simulink model "sampleModel1955_4_sub"  (R2023a)
settings: Solver=VariableStepAuto  StartTime=0.0  StopTime=10.0  RelTol=1e-3
libraries: simulink x6, hdlsllib x4
settings Model: Creator=user1  LastModifiedBy=user1
settings OptimizationCC: BlockReduction=off  ConditionallyExecuteInputs=off

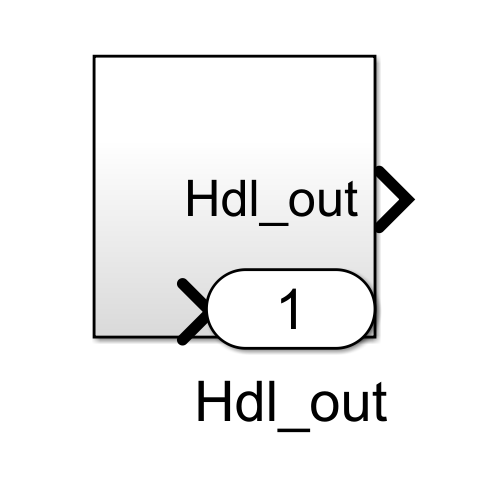
[thumbnail: Simulink's stored preview of the top-level diagram]
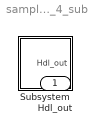
== system sampleModel1955_4_sub ==
  Subsystem : Subsystem
  Hdl_out : Outport  OutDataTypeStr=uint8

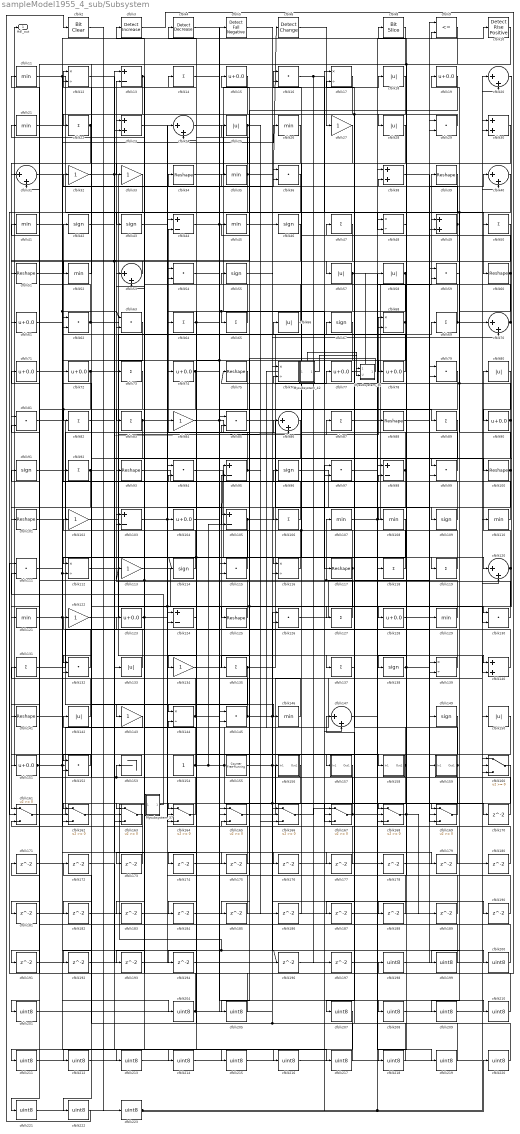
== system sampleModel1955_4_sub/Subsystem ==
  Mysubsystem_30 : Subsystem  TreatAsAtomicUnit=on  RTWFcnName=Mysubsystem_30
      settings: RTWFcnNameOpts=User specified  RTWFileNameOpts=Use function name
  Mysubsystem_37 : Subsystem  TreatAsAtomicUnit=on  RTWFcnName=Mysubsystem_37
      settings: RTWFcnNameOpts=User specified  RTWFileNameOpts=Use function name
  Mysubsystem_42 : Subsystem  TreatAsAtomicUnit=on  RTWFcnName=Mysubsystem_42
      settings: RTWFcnNameOpts=User specified  RTWFileNameOpts=Use function name
  cfblk10 : hdlsllib/Logic and Bit Operations/Detect Rise Positive  vinit=0  OutDataTypeStr=uint8
  cfblk{34,39,51,60,75,88,93,100..101,117,125,141} (12 alike) : Reshape
  cfblk{27,32..33,84,102,113,122,134,143} (9 alike) : Gain  OutDataTypeStr=uint8
  cfblk{13,44,95,98,103,105,124} (7 alike) : Sum  Inputs=+-  OutDataTypeStr=uint8
  cfblk{15,19,61,71..72,74,77..78,90,104,123,128,151} (13 alike) : Bias  Bias=0.0  SaturateOnIntegerOverflow=off
  cfblk{14,22,47,50,64..65,69,73,82..83,87,89,92,106,118..119,127,131,135,137} (20 alike) : Sum  Inputs=+  OutDataTypeStr=uint8
  cfblk{11,21,26,35,41,45,52,107..108,110,121,129,146} (13 alike) : MinMax  OutDataTypeStr=uint8
  cfblk{42..43,46,55,67,91,96,109,114,138,149} (11 alike) : Signum
  cfblk{16,29,36,54,59,62..63,79,81,85,94,97,99,111,115,126,130,132,145,152} (20 alike) : DotProduct  OutDataTypeStr=uint8
  cfblk{12,17,48,68,76,112,116,139,144} (9 alike) : Product  Inputs=*/  OutDataTypeStr=uint8  RndMeth=Zero  SaturateOnIntegerOverflow=on
  cfblk{20,24,31,40,53,70,86,120,147} (9 alike) : Sum  Inputs=|++  OutDataTypeStr=uint8
  cfblk{18,25,28,57..58,66,80,133,142,150} (10 alike) : Abs  OutDataTypeStr=uint8  SaturateOnIntegerOverflow=off
  cfblk{23,30,38,49,140} (5 alike) : Sum  OutDataTypeStr=uint8
  cfblk153 : Terminator
  cfblk154 : Constant  OutDataTypeStr=uint8  SampleTime=-1
  cfblk155 : hdlsllib/Sources/Counter Free-Running  NumBits=16  tsamp=-1
  cfblk156 : Subsystem
      settings: LibrarySourceBlock=|
      | hdlsllib/Ports &
      | Subsystems/Subsystem
  cfblk157 : Subsystem
      settings: LibrarySourceBlock=|
      | hdlsllib/Ports &
      | Subsystems/Subsystem
  cfblk158 : Subsystem
      settings: LibrarySourceBlock=|
      | hdlsllib/Ports &
      | Subsystems/Subsystem
  cfblk159 : Subsystem
      settings: LibrarySourceBlock=|
      | hdlsllib/Ports &
      | Subsystems/Subsystem
  cfblk{160..169} (10 alike) : Switch  OutDataTypeStr=uint8  SaturateOnIntegerOverflow=off  InputSameDT=off
  cfblk{170..194,196..197} (27 alike) : Delay  SampleTime=1
  cfblk{198..201,204..205,207..223} (23 alike) : DataTypeConversion  OutDataTypeStr=uint8  SaturateOnIntegerOverflow=off  RndMeth=Floor
  cfblk2 : simulink/Logic and Bit Operations/Bit Clear  iBit=0
      settings: LibrarySourceBlock=|
      | hdlsllib/Logic and Bit
      | Operations/Bit Clear
  cfblk3 : simulink/Logic and Bit Operations/Detect Increase  vinit=0.0  OutDataTypeStr=uint8
      settings: LibrarySourceBlock=|
      | hdlsllib/Logic and Bit
      | Operations/Detect
      | Increase
  cfblk4 : simulink/Logic and Bit Operations/Detect Decrease  vinit=0.0  OutDataTypeStr=uint8
      settings: LibrarySourceBlock=|
      | hdlsllib/Logic and Bit
      | Operations/Detect
      | Decrease
  cfblk5 : hdlsllib/Logic and Bit Operations/Detect Fall Negative  vinit=0  OutDataTypeStr=uint8
  cfblk6 : simulink/Logic and Bit Operations/Detect Change  vinit=0  OutDataTypeStr=uint8
      settings: LibrarySourceBlock=|
      | hdlsllib/Logic and Bit
      | Operations/Detect
      | Change
  cfblk8 : hdlsllib/Logic and Bit Operations/Bit Slice  lidx=7  ridx=0
  cfblk9 : RelationalOperator  Operator=<=  OutDataTypeStr=boolean  InputSameDT=off
  Hdl_out : Outport  OutDataTypeStr=uint8
  wires:
  cfblk81/1 -> cfblk143/1
  cfblk29/1 -> cfblk28/1
  cfblk77/1 -> cfblk58/1
  cfblk144/1 -> cfblk179/1, cfblk102/1
  cfblk135/1 -> cfblk162/1, cfblk77/1
  cfblk92/1 -> cfblk191/1, cfblk100/1
  cfblk143/1 -> cfblk142/1
  cfblk19/1 -> cfblk161/1
  cfblk105/1 -> cfblk69/1, cfblk184/1, cfblk114/1
  cfblk83/1 -> cfblk192/1, cfblk67/1
  cfblk20/1 -> cfblk99/1
  cfblk95/1 -> cfblk186/1, cfblk44/2
  cfblk26/1 -> cfblk81/1
  cfblk164/1 -> cfblk122/1
  cfblk127/1 -> cfblk34/1, cfblk107/1
  cfblk32/1 -> cfblk86/2, cfblk137/1
  cfblk107/1 -> cfblk9/2, cfblk39/1
  cfblk6/1 -> cfblk27/1
  cfblk122/1 -> cfblk66/1
  cfblk106/1 -> cfblk42/1
  cfblk27/1 -> cfblk106/1
  cfblk48/1 -> cfblk138/1
  cfblk130/1 -> cfblk13/2
  cfblk169/1 -> cfblk91/1
  cfblk57/1 -> cfblk169/2, cfblk164/2, cfblk65/1
  cfblk96/1 -> cfblk139/2
  cfblk34/1 -> cfblk18/1
  cfblk73/1 -> cfblk101/1, cfblk82/1
  cfblk44/1 -> cfblk140/1, cfblk76/1
  cfblk28/1 -> cfblk33/1
  cfblk9/1 -> cfblk218/1, cfblk212/1
  cfblk161/1 -> cfblk118/1
  cfblk116/1 -> cfblk72/1
  cfblk112/1 -> cfblk87/1
  cfblk45/1 -> cfblk46/1
  cfblk162/1 -> cfblk73/1
  cfblk113/1 -> cfblk128/1
  cfblk94/1 -> cfblk120/1
  cfblk43/1 -> cfblk124/1
  cfblk101/1 -> cfblk17/1
  cfblk147/1 -> cfblk219/1
  cfblk25/1 -> cfblk166/3, cfblk61/1
  cfblk151/1 -> Hdl_out/1, cfblk36/2, cfblk133/1
  cfblk90/1 -> cfblk199/1, cfblk49/1, cfblk75/1
  cfblk10/1 -> cfblk52/1
  cfblk24/1 -> cfblk117/1
  cfblk35/1 -> cfblk221/1, cfblk12/2, cfblk6/1
  cfblk74/1 -> cfblk201/1, cfblk157/1(In1)
  cfblk49/1 -> cfblk12/1, cfblk108/1
  cfblk118/1 -> cfblk76/2, cfblk95/1
  cfblk168/1 -> cfblk189/1, cfblk188/1
  cfblk2/1 -> cfblk223/1
  cfblk120/1 -> cfblk164/3, cfblk80/1
  cfblk137/1 -> cfblk17/2
  cfblk11/1 -> cfblk216/1, cfblk60/1
  cfblk36/1 -> cfblk163/1
  cfblk140/1 -> cfblk14/1
  cfblk89/1 -> cfblk116/1
  cfblk78/1 -> cfblk15/1
  cfblk121/1 -> cfblk35/1, cfblk196/1, Mysubsystem_37/1(In1)
  cfblk91/1 -> cfblk74/1
  cfblk134/1 -> cfblk95/2
  cfblk129/1 -> cfblk47/1
  cfblk123/1 -> cfblk127/1, cfblk23/1
  cfblk50/1 -> cfblk57/1
  cfblk117/1 -> cfblk53/1, cfblk132/1, cfblk135/1
  cfblk84/1 -> cfblk177/1, cfblk86/1
  cfblk110/1 -> cfblk54/1
  cfblk23/1 -> cfblk105/1
  cfblk39/1 -> cfblk161/2
  cfblk18/1 -> cfblk187/1, cfblk132/2
  cfblk62/1 -> cfblk31/2, cfblk85/1
  cfblk146/1 -> cfblk53/2
  cfblk40/1 -> cfblk49/2, cfblk169/1
  cfblk17/1 -> cfblk22/1
  cfblk159/1(Out1) -> cfblk168/2, cfblk93/1
  cfblk22/1 -> cfblk182/1, cfblk181/1
  cfblk154/1 -> cfblk113/1, cfblk103/1, cfblk105/2, cfblk169/3, Mysubsystem_42/1(In1)
  cfblk38/1 -> cfblk159/1(In1)
  cfblk52/1 -> cfblk32/1
  cfblk87/1 -> cfblk29/1
  cfblk128/1 -> cfblk149/1
  cfblk93/1 -> cfblk98/2
  cfblk155/1 -> cfblk167/3, cfblk168/1
  cfblk138/1 -> cfblk170/1, cfblk38/2
  cfblk99/1 -> cfblk68/1
  cfblk55/1 -> cfblk70/2
  cfblk47/1 -> cfblk163/2, cfblk121/1
  cfblk59/1 -> cfblk109/1
  cfblk145/1 -> cfblk123/1, cfblk79/2, cfblk190/1, cfblk168/3
  cfblk53/1 -> cfblk51/1
  cfblk131/1 -> cfblk29/2
  cfblk46/1 -> cfblk145/2
  cfblk156/1(Out1) -> cfblk165/2
  cfblk58/1 -> cfblk194/1, cfblk78/1
  cfblk69/1 -> cfblk40/2, cfblk8/1
  cfblk165/1 -> cfblk20/1
  cfblk163/1 -> cfblk161/3
  cfblk100/1 -> cfblk19/1, cfblk152/1
  cfblk115/1 -> cfblk24/2
  cfblk158/1(Out1) -> cfblk162/2, cfblk64/1
  cfblk64/1 -> cfblk140/2, cfblk4/1
  cfblk51/1 -> cfblk152/2
  cfblk65/1 -> cfblk55/1
  cfblk139/1 -> cfblk45/1
  cfblk60/1 -> cfblk209/1, cfblk36/1
  cfblk68/1 -> cfblk134/1, cfblk16/1
  cfblk102/1 -> cfblk124/2
  cfblk167/1 -> cfblk59/2, cfblk92/1, cfblk153/1
  cfblk72/1 -> cfblk119/1, cfblk141/1
  cfblk141/1 -> cfblk94/2
  cfblk132/1 -> cfblk11/1
  cfblk125/1 -> cfblk41/1
  cfblk13/1 -> cfblk23/2, cfblk83/1
  cfblk33/1 -> cfblk43/1
  cfblk14/1 -> cfblk89/1
  cfblk111/1 -> cfblk204/1
  cfblk108/1 -> cfblk112/1
  cfblk66/1 -> cfblk21/1
  cfblk42/1 -> cfblk50/1
  cfblk71/1 -> cfblk10/1
  cfblk82/1 -> cfblk144/1
  cfblk85/1 -> cfblk129/1
  cfblk133/1 -> cfblk81/2
  cfblk109/1 -> cfblk96/1
  cfblk79/1 -> cfblk125/1
  cfblk41/1 -> cfblk116/2
  cfblk70/1 -> cfblk130/1, cfblk25/1
  cfblk88/1 -> cfblk40/1
  cfblk80/1 -> cfblk90/1
  cfblk8/1 -> cfblk31/1
  cfblk103/1 -> cfblk104/1, cfblk130/2, cfblk146/1
  cfblk104/1 -> cfblk88/1
  cfblk152/1 -> cfblk151/1
  cfblk119/1 -> cfblk84/1
  cfblk54/1 -> cfblk126/2
  cfblk61/1 -> cfblk26/1
  cfblk16/1 -> cfblk197/1, cfblk48/2
  cfblk166/1 -> cfblk167/1
  cfblk31/1 -> cfblk158/1(In1), cfblk63/1
  cfblk67/1 -> cfblk115/2, cfblk164/1
  cfblk126/1 -> cfblk9/1
  cfblk114/1 -> cfblk63/2
  cfblk142/1 -> cfblk131/1
  cfblk63/1 -> cfblk162/3, cfblk112/2
  cfblk98/1 -> cfblk163/3, cfblk62/2
  cfblk170/1 -> cfblk48/1
  cfblk75/1 -> cfblk173/1
  cfblk173/1 -> cfblk62/1
  cfblk150/1 -> cfblk174/1
  cfblk174/1 -> cfblk167/2
  cfblk12/1 -> cfblk175/1
  cfblk175/1 -> cfblk94/1
  cfblk21/1 -> cfblk176/1
  cfblk176/1 -> cfblk120/2
  cfblk177/1 -> cfblk165/1
  cfblk178/1 -> cfblk79/1
  cfblk179/1 -> cfblk139/1
  cfblk180/1 -> cfblk165/3
  cfblk181/1 -> cfblk59/1
  cfblk182/1 -> cfblk166/2
  cfblk157/1(Out1) -> cfblk183/1
  cfblk183/1 -> cfblk98/1
  cfblk184/1 -> cfblk166/1
  cfblk185/1 -> cfblk44/1
  cfblk186/1 -> cfblk16/2
  cfblk187/1 -> cfblk38/1
  cfblk188/1 -> cfblk145/1
  cfblk189/1 -> cfblk68/2
  cfblk190/1 -> cfblk85/2
  cfblk191/1 -> cfblk70/1
  cfblk192/1 -> cfblk13/1
  cfblk15/1 -> cfblk193/1
  cfblk193/1 -> cfblk24/1
  cfblk194/1 -> cfblk115/1
  cfblk196/1 -> cfblk20/2
  cfblk197/1 -> cfblk99/2
  cfblk3/1 -> cfblk198/1
  cfblk198/1 -> cfblk150/1
  cfblk199/1 -> cfblk3/1
  cfblk5/1 -> cfblk200/1
  cfblk200/1 -> cfblk71/1
  cfblk201/1 -> cfblk5/1
  cfblk204/1 -> cfblk156/1(In1), cfblk103/2
  cfblk149/1 -> cfblk205/1
  cfblk205/1 -> cfblk111/1
  cfblk30/1 -> cfblk207/1
  cfblk4/1 -> cfblk208/1
  cfblk208/1 -> cfblk30/1
  cfblk209/1 -> cfblk30/2
  cfblk97/1 -> cfblk210/1
  cfblk210/1 -> cfblk171/1
  cfblk207/1 -> cfblk211/1
  cfblk211/1 -> cfblk97/1
  cfblk212/1 -> cfblk97/2
  cfblk160/1 -> cfblk213/1
  cfblk213/1 -> cfblk110/1
  cfblk124/1 -> cfblk214/1
  cfblk214/1 -> cfblk160/1
  cfblk171/1 -> cfblk215/1
  cfblk215/1 -> cfblk160/2
  cfblk216/1 -> cfblk160/3
  cfblk172/1 -> cfblk217/1
  cfblk217/1 -> cfblk54/2
  cfblk218/1 -> cfblk172/1
  cfblk219/1 -> cfblk126/1, cfblk144/2
  cfblk220/1 -> cfblk147/1
  cfblk221/1 -> cfblk147/2
  cfblk86/1 -> cfblk222/1
  cfblk222/1 -> cfblk2/1
  cfblk223/1 -> cfblk220/1, cfblk178/1, cfblk180/1
  cfblk76/1 -> Mysubsystem_30/2(U)
  Mysubsystem_30/1(Out1) -> cfblk185/1
  Mysubsystem_37/1(Out1) -> cfblk111/2
  Mysubsystem_42/1(Out1) -> Mysubsystem_30/1(In1)

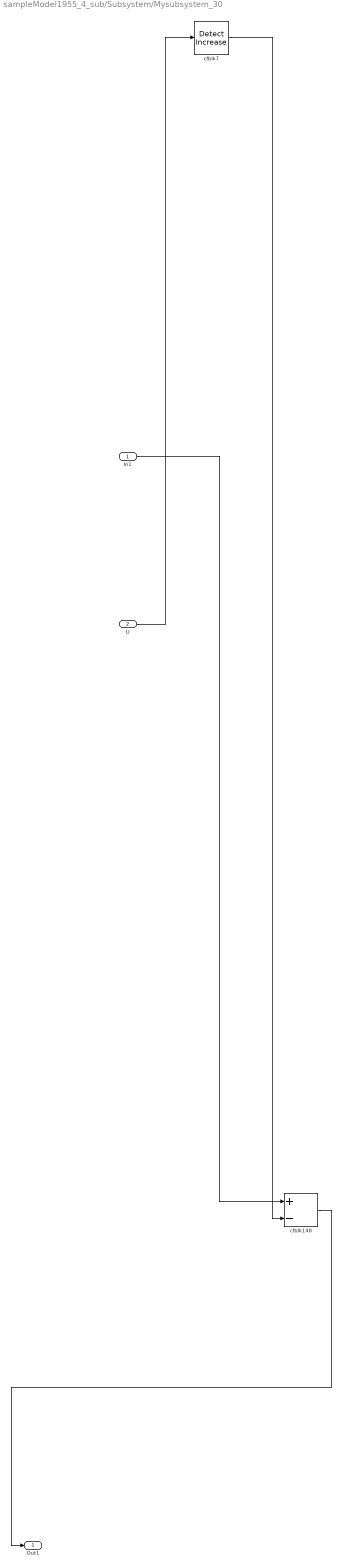
== system sampleModel1955_4_sub/Subsystem/Mysubsystem_30 ==
  In1 : Inport
  U : Inport  Port=2
  cfblk148 : Sum  Inputs=+-
  cfblk7 : simulink/Logic and Bit Operations/Detect Increase  vinit=0.0  OutDataTypeStr=boolean
      settings: LibrarySourceBlock=|
      | hdlsllib/Logic and Bit
      | Operations/Detect
      | Increase
  Out1 : Outport
  wires:
  U/1 -> cfblk7/1
  In1/1 -> cfblk148/1
  cfblk7/1 -> cfblk148/2
  cfblk148/1 -> Out1/1

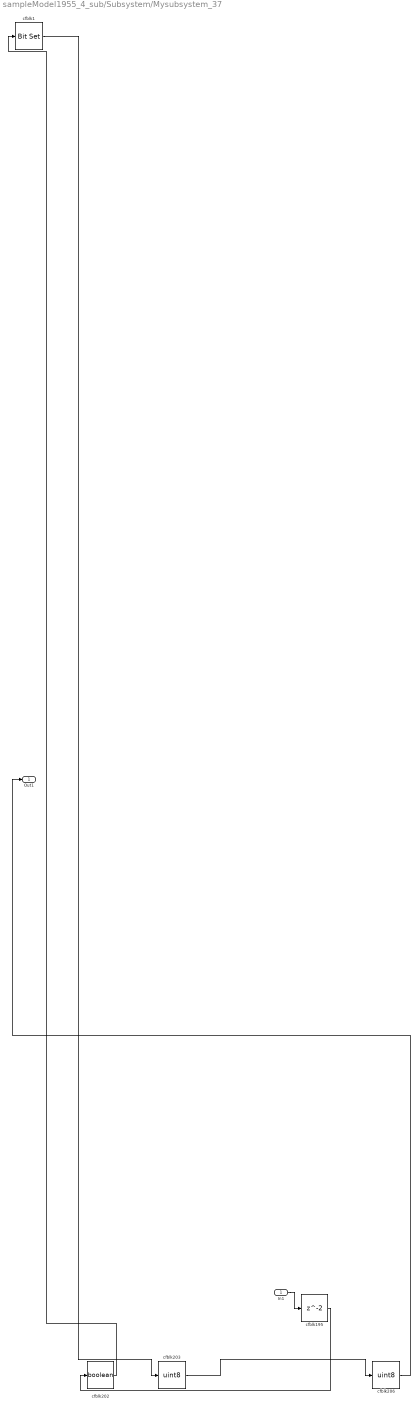
== system sampleModel1955_4_sub/Subsystem/Mysubsystem_37 ==
  In1 : Inport
  cfblk1 : simulink/Logic and Bit Operations/Bit Set  iBit=0
      settings: LibrarySourceBlock=|
      | hdlsllib/Logic and Bit
      | Operations/Bit Set
  cfblk195 : Delay  SampleTime=1
  cfblk202 : DataTypeConversion  OutDataTypeStr=boolean  SaturateOnIntegerOverflow=off  RndMeth=Floor
  cfblk203 : DataTypeConversion  OutDataTypeStr=uint8  SaturateOnIntegerOverflow=off  RndMeth=Floor
  cfblk206 : DataTypeConversion  OutDataTypeStr=uint8  SaturateOnIntegerOverflow=off  RndMeth=Floor
  Out1 : Outport
  wires:
  In1/1 -> cfblk195/1
  cfblk203/1 -> cfblk206/1
  cfblk1/1 -> cfblk203/1
  cfblk202/1 -> cfblk1/1
  cfblk206/1 -> Out1/1
  cfblk195/1 -> cfblk202/1

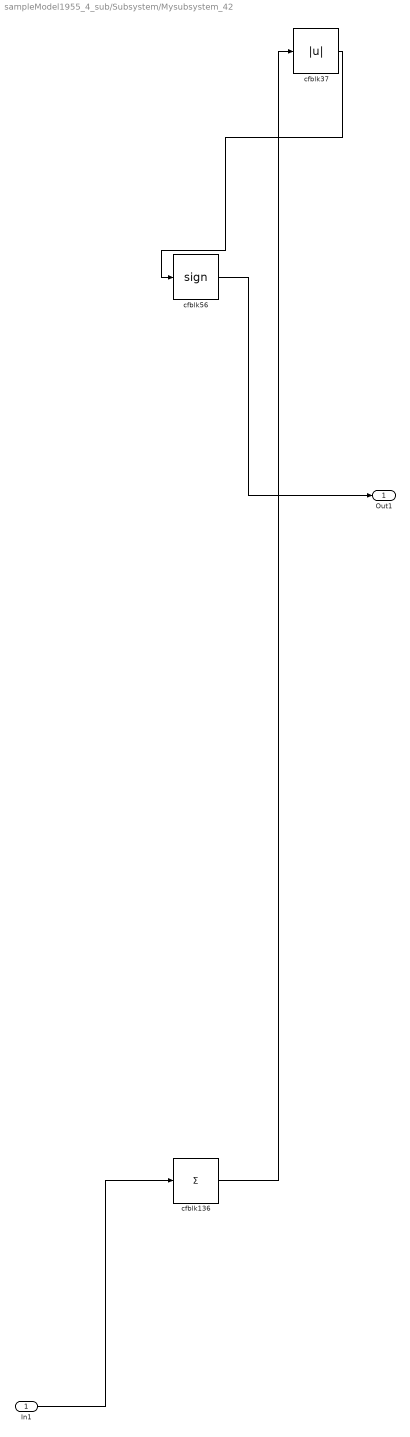
== system sampleModel1955_4_sub/Subsystem/Mysubsystem_42 ==
  In1 : Inport
  cfblk136 : Sum  Inputs=+
  cfblk37 : Abs  SaturateOnIntegerOverflow=off
  cfblk56 : Signum
  Out1 : Outport
  wires:
  cfblk56/1 -> Out1/1
  In1/1 -> cfblk136/1
  cfblk136/1 -> cfblk37/1
  cfblk37/1 -> cfblk56/1

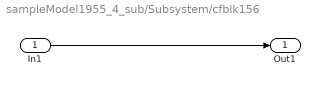
== system sampleModel1955_4_sub/Subsystem/cfblk156 ==
  In1 : Inport
  Out1 : Outport
  wires:
  In1/1 -> Out1/1

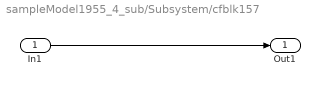
== system sampleModel1955_4_sub/Subsystem/cfblk157 ==
  In1 : Inport
  Out1 : Outport
  wires:
  In1/1 -> Out1/1

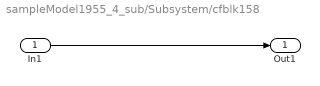
== system sampleModel1955_4_sub/Subsystem/cfblk158 ==
  In1 : Inport
  Out1 : Outport
  wires:
  In1/1 -> Out1/1

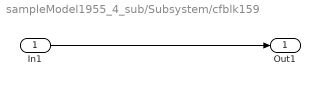
== system sampleModel1955_4_sub/Subsystem/cfblk159 ==
  In1 : Inport
  Out1 : Outport
  wires:
  In1/1 -> Out1/1
